simulink model "reg_and_object"  (R2018a)
settings: Solver=VariableStepAuto  StartTime=0.0  StopTime=100  MaxStep=1e-2  RelTol=1e-3
values from neighbouring files (symbols this model uses):
  B = 1    [data.m]
  C = 5    [data.m]
  kD = kD1    (= 0)    [data.m]
  kI = kI1    (= 23.4784)    [data.m]
  kP = kP1    (= 4.6957)    [data.m]
  V1 = 10    [data.m]
  V2 = 20    [data.m]
  yref = 50    [data.m]
libraries: simulink x1
settings Model: Creator=User  LastModifiedBy=User
settings OptimizationCC: DefaultParameterBehavior=Inlined  UseDivisionForNetSlopeComputation=on  UseFloatMulNetSlope=on  InlineInvariantSignals=on  PassReuseOutputArgsAs=Individual arguments  ZeroExternalMemoryAtStartup=off  ZeroInternalMemoryAtStartup=off  NoFixptDivByZeroProtection=on  EfficientFloat2IntCast=on  LifeSpan=1  OptimizeBlockOrder=speed  DifferentSizesBufferReuse=on
settings DebuggingCC: ParameterTunabilityLossMsg=error
settings HardwareCC: ProdLongLongMode=on
settings SFSimCC: MATLABDynamicMemAlloc=off
settings RTWCC: SystemTargetFile=ert.tlc  TemplateMakefile=ert_default_tmf  GenerateReport=on  IncludeHyperlinkInReport=on  LaunchReport=on  GenerateTraceInfo=on  GenerateTraceReport=on  GenerateTraceReportSl=on  GenerateTraceReportSf=on  GenerateTraceReportEml=on  GenerateCodeMetricsReport=on
settings CodeAppCC: ForceParamTrailComments=on  IgnoreCustomStorageClasses=off  OperatorAnnotations=on  SimulinkDataObjDesc=on  SFDataObjDesc=on  CustomSymbolStrGlobalVar=rt$N$M  CustomSymbolStrType=$N$M  CustomSymbolStrFcn=$N$M$F  CustomSymbolStrMacro=$N$M  InsertBlockDesc=on
settings ERTTargetCC: TargetLangStandard=C99 (ISO)  GenerateSampleERTMain=on  IncludeMdlTerminateFcn=off  CombineSignalStateStructs=on  SupportAbsoluteTime=off  SupportComplex=off  InlinedParameterPlacement=NonHierarchical  ERTCustomFileTemplate=example_file_process.tlc  ERTFilePackagingFormat=CompactWithDataFile

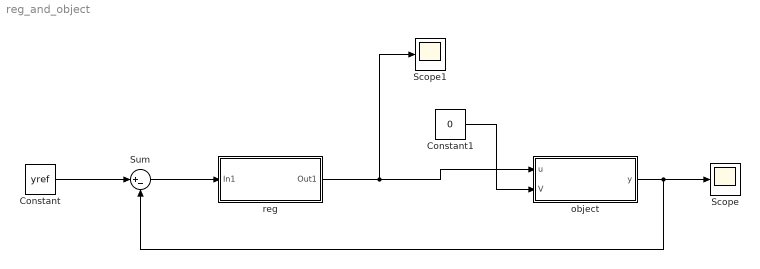
== system reg_and_object ==
  Constant : Constant  Value=yref
  Constant1 : Constant  Value=0
  Scope : Scope
  Scope1 : Scope
  Sum : Sum  Inputs=|+-
  object : Subsystem
  reg : Subsystem
  wires:
  reg/1(Out1) -> Scope1/1, object/1(u)
  object/1(y) -> Scope/1, Sum/2
  Sum/1 -> reg/1(In1)
  Constant/1 -> Sum/1
  Constant1/1 -> object/2(V)

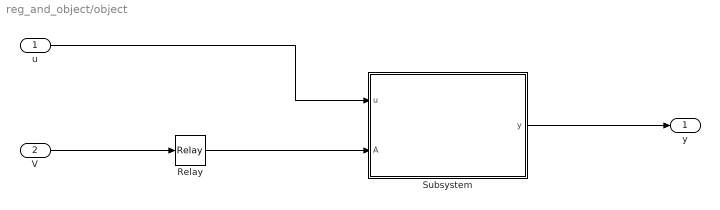
== system reg_and_object/object ==
  u : Inport
  V : Inport  Port=2
  Relay : Relay  OnSwitchValue=V2  OffSwitchValue=V1  OnOutputValue=A2  OffOutputValue=A1
  Subsystem : Subsystem
  y : Outport
  wires:
  V/1 -> Relay/1
  Relay/1 -> Subsystem/2(A)
  u/1 -> Subsystem/1(u)
  Subsystem/1(y) -> y/1

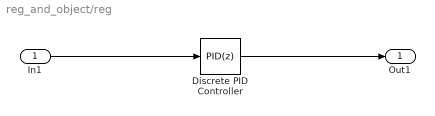
== system reg_and_object/reg ==
  In1 : Inport
  Discrete PID Controller : simulink/Continuous/PID Controller  Controller=PID  TimeDomain=Discrete-time  SampleTime=0.01  IntegratorMethod=Forward Euler  FilterMethod=Forward Euler  Form=Parallel  UseFilter=on  ControllerParametersSource=internal  P=kP  I=kI  D=kD  N=53.7209719437635  InitialConditionSource=internal  InitialConditionForIntegrator=0  InitialConditionForFilter=0  ExternalReset=none  LimitOutput=off  UpperSaturationLimit=inf  LowerSaturationLimit=-inf  LinearizeAsGain=off  AntiWindupMode=none  Kb=1  TrackingMode=off  Kt=1  PParamMin=[]  PParamMax=[]  IParamMin=[]  IParamMax=[]  DParamMin=[]  DParamMax=[]  NParamMin=[]  NParamMax=[]  KbParamMin=[]  KbParamMax=[]  KtParamMin=[]  KtParamMax=[]  POutMin=[]  POutMax=[]  IOutMin=[]  IOutMax=[]  DOutMin=[]  DOutMax=[]  NOutMin=[]  NOutMax=[]  KbOutMin=[]  KbOutMax=[]  KtOutMin=[]  KtOutMax=[]  IntegratorOutMin=[]  IntegratorOutMax=[]  FilterOutMin=[]  FilterOutMax=[]  SumOutMin=[]  SumOutMax=[]  SumI1OutMin=[]  SumI1OutMax=[]  SumI2OutMin=[]  SumI2OutMax=[]  SumI3OutMin=[]  SumI3OutMax=[]  SumDOutMin=[]  SumDOutMax=[]  SaturationOutMin=[]  SaturationOutMax=[]  IntegratorContinuousStateAttributes=''  IntegratorStateMustResolveToSignalObject=off  IntegratorRTWStateStorageClass=Auto  FilterContinuousStateAttributes=''  FilterStateMustResolveToSignalObject=off  FilterRTWStateStorageClass=Auto  DifferentiatorICPrevScaledInput=0  DifferentiatorOutMin=[]  DifferentiatorOutMax=[]  FilterDiffOutCoefMin=[]  FilterDiffOutCoefMax=[]  SumDenOutMin=[]  SumDenOutMax=[]  SumNumOutMin=[]  SumNumOutMax=[]  ReciprocalOutMin=[]  ReciprocalOutMax=[]  DivideOutMin=[]  DivideOutMax=[]  TunerSelectOption=Transfer Function Based (PID Tuner App)
  Out1 : Outport
  wires:
  In1/1 -> Discrete PID Controller/1
  Discrete PID Controller/1 -> Out1/1

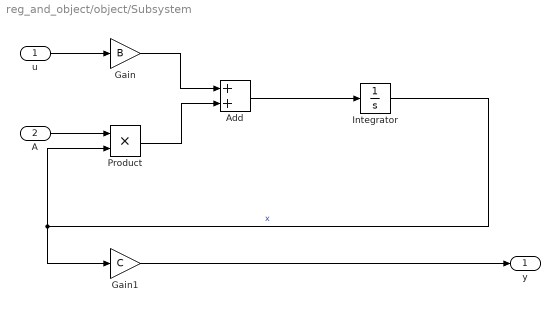
== system reg_and_object/object/Subsystem ==
  u : Inport
  A : Inport  Port=2
  Add : Sum
  Gain : Gain  Gain=B
  Gain1 : Gain  Gain=C
  Integrator : Integrator
  Product : Product
  y : Outport
  wires:
  A/1 -> Product/1
  Integrator/1 -> Gain1/1, Product/2  "x"
  u/1 -> Gain/1
  Gain/1 -> Add/1
  Product/1 -> Add/2
  Add/1 -> Integrator/1
  Gain1/1 -> y/1
